simulink model "sistema_furuta"  (R2024a)
settings: Solver=VariableStepAuto  StartTime=0.0  StopTime=10.0  RelTol=1e-3
settings Model: SimulationMode=accelerator  Creator=PC  LastModifiedBy=PC
settings RTWCC: GPUComputeCapability=3.5

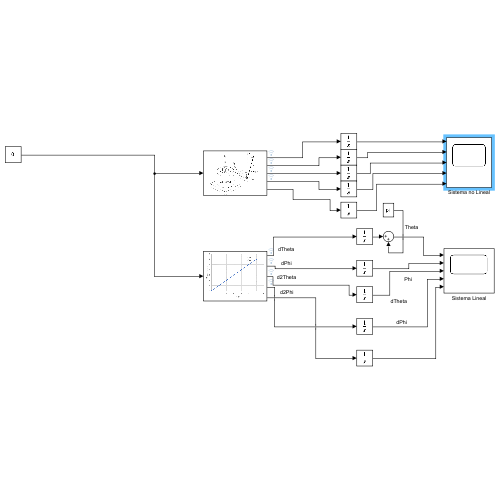
[thumbnail: Simulink's stored preview of the top-level diagram]
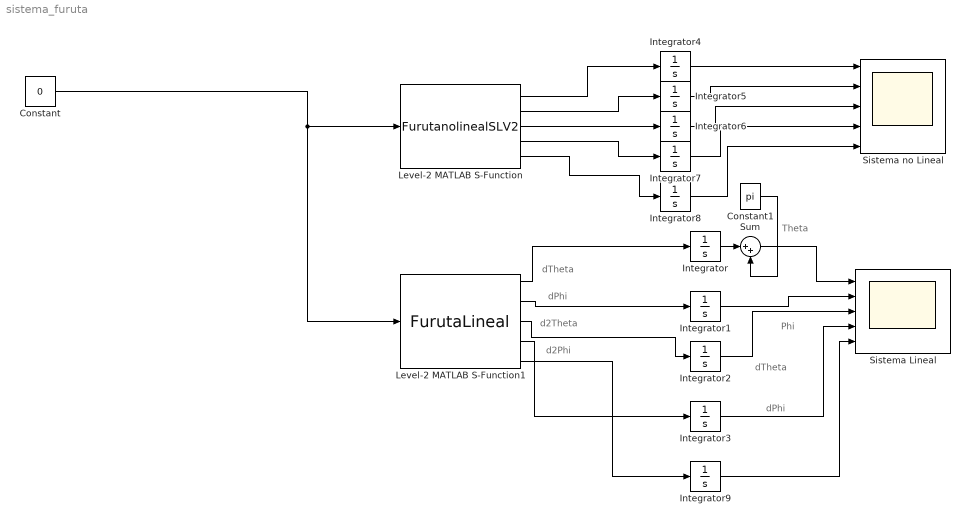
== system sistema_furuta ==
  note: dPhi
  note: dTheta
  note: Phi
  note: Theta
  note: d2Phi
  note: d2Theta
  note: dPhi
  note: dTheta
  Constant : Constant  Value=0
  Constant1 : Constant  Value=pi
  Integrator : Integrator  InitialCondition=pi
  Integrator{1..9} (9 alike) : Integrator
  Level-2 MATLAB S-Function : M-S-Function  FunctionName=FurutanolinealSLV2  mask{Xi=0, g=0, J=0, M_2=0, l_bi=0, C_x=0, C_z=0, I_x=0, I_z=0}
      mask prompts: Xi "Parametros iniciales (Xi)"
      mask Display: image('mascara2.png');
  Level-2 MATLAB S-Function1 : M-S-Function  FunctionName=FurutaLineal  mask{Xi=0, g=0, J=0, M_2=0, l_bi=0, C_x=0, C_z=0, I_x=0, I_z=0}
      mask prompts: Xi "Parametros iniciales (Xi)"
      mask Display: image('Lineal.png');
  Sistema Lineal : Scope  NumInputPorts=5
  Sistema no Lineal : Scope  NumInputPorts=5
  Sum : Sum  Inputs=|++
  wires:
  Level-2 MATLAB S-Function/1 -> Integrator4/1
  Level-2 MATLAB S-Function1/2 -> Integrator1/1
  Level-2 MATLAB S-Function1/3 -> Integrator2/1
  Level-2 MATLAB S-Function1/4 -> Integrator3/1
  Level-2 MATLAB S-Function/2 -> Integrator5/1
  Level-2 MATLAB S-Function/3 -> Integrator6/1
  Level-2 MATLAB S-Function/4 -> Integrator7/1
  Constant/1 -> Level-2 MATLAB S-Function1/1, Level-2 MATLAB S-Function/1
  Level-2 MATLAB S-Function1/1 -> Integrator/1
  Integrator/1 -> Sum/1
  Constant1/1 -> Sum/2
  Sum/1 -> Sistema Lineal/1
  Integrator1/1 -> Sistema Lineal/2
  Integrator2/1 -> Sistema Lineal/3
  Integrator3/1 -> Sistema Lineal/4
  Integrator4/1 -> Sistema no Lineal/1
  Integrator5/1 -> Sistema no Lineal/2
  Integrator6/1 -> Sistema no Lineal/3
  Integrator7/1 -> Sistema no Lineal/4
  Level-2 MATLAB S-Function/5 -> Integrator8/1
  Integrator8/1 -> Sistema no Lineal/5
  Integrator9/1 -> Sistema Lineal/5
  Level-2 MATLAB S-Function1/5 -> Integrator9/1
